simulink model "Implantation_Cmd_MCC_PI"  (R2018b)
settings: Solver=ode1  StartTime=0.0  StopTime=15  FixedStep=Te1  RelTol=1e-3  EnableMultiTasking=on
values from neighbouring files (symbols this model uses):
  Te1 = 0.002    [InitCommande_Aero.m]    (also in matlab_variables_2_2.mat)
undefined symbols (not defined in the file or in its folder): Kpw, Tiw
libraries: quanser_aero x1, simulink_extras x1
settings Model: SimulationMode=external  ExtModeTrigDuration=50000  Creator=MLevis  LastModifiedBy=ACS3
settings SolverCC: PositivePriorityOrder=on
settings DataIOCC: SaveFormat=Array  DSMLogging=off
settings OptimizationCC: LifeSpan=inf
settings DebuggingCC: SolverPrmCheckMsg=warning  SFUnexpectedBacktrackingDiag=warning  SFNoUnconditionalDefaultTransitionDiag=warning  SFExecutionAtInitializationDiag=none
settings HardwareCC: ProdBitPerPointer=32  ProdBitPerSizeT=32  ProdBitPerPtrDiffT=32  ProdLargestAtomicFloat=None  ProdIntDivRoundTo=Undefined  ProdEndianess=Unspecified  ProdWordSize=32  ProdHWDeviceType=32-bit Generic
settings ModelReferenceCC: PropagateSignalLabelsOutOfModel=off
settings SFSimCC: SimUseLocalCustomCode=off
settings RTWCC: SystemTargetFile=quarc_win64.tlc  TemplateMakefile=quarc_default_tmf  Description=QUARC Win64 Target  RTWUseLocalCustomCode=off
settings CodeAppCC: StateflowObjectComments=on
settings STFCustomTargetCC: TargetPreCompLibLocation=C:\PROGRA~3\QUARC\lib\2018b\win64\release  ConcurrentExecutionCompliant=on  GeneratePreprocessorConditionals=Disable all  GRTInterface=on  SystemTargetFile=quarc_win64.tlc
settings GRTTargetCC: TargetPreCompLibLocation=C:\PROGRA~3\QUARC\lib\2018b\win64\release  TargetLangStandard=C89/C90 (ANSI)  ParMdlRefBuildCompliant=off  CompOptLevelCompliant=off  GeneratePreprocessorConditionals=Disable all  CombineOutputUpdateFcns=off  MatFileLogging=off  CPPClassGenCompliant=off  GRTInterface=on  UseToolchainInfoCompliant=off  ExtMode=on  ExtModeMexFile=quarc_comm
settings ConfigComp: CovMetricSettings=dw  CovHtmlReporting=on  CovSaveCumulativeToWorkspaceVar=on  CovSaveSingleToWorkspaceVar=on  CovExternalEMLEnable=off  CovSFcnEnable=off

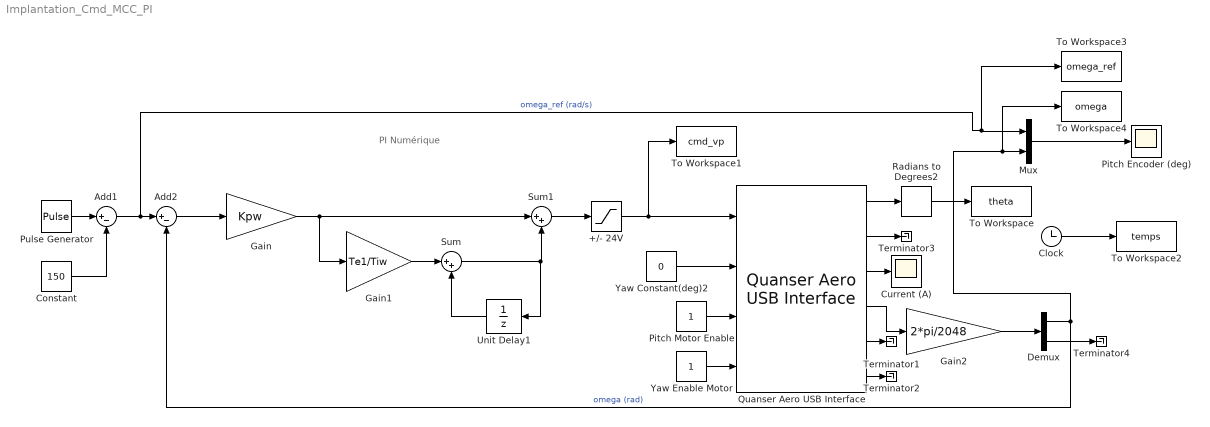
== system Implantation_Cmd_MCC_PI ==
  note: PI Numérique
  +/- 24V : Saturate  UpperLimit=24  LowerLimit=-24
  Add1 : Sum  Inputs=|+-
  Add2 : Sum  Inputs=|+-
  Clock : Clock
  Constant : Constant  Value=150
  Current (A) : Scope
  Demux : Demux  Outputs=2
  Gain : Gain  Gain=Kpw
  Gain1 : Gain  Gain=Te1/Tiw
  Gain2 : Gain  Gain=2*pi/2048
  Mux : Mux  Inputs=2
  Pitch Encoder (deg) : Scope
  Pitch Motor Enable : Constant
  Pulse Generator : DiscretePulseGenerator  PulseType=Time based  Amplitude=150*2  Period=6  PulseWidth=50
  Quanser Aero USB Interface : quanser_aero/Quanser Aero USB Interface  SystemSampleTime=-1
  Radians to Degrees2 : simulink_extras/Transformations/Radians to Degrees
  Sum : Sum  Inputs=|++
  Sum1 : Sum  Inputs=|++
  Terminator{1..4} (4 alike) : Terminator
  To Workspace : ToWorkspace  VariableName=theta  SampleTime=-1
      settings: Save2DSignal=2-D array (concatenate along first dimension)
  To Workspace1 : ToWorkspace  VariableName=cmd_vp  SampleTime=-1
      settings: Save2DSignal=2-D array (concatenate along first dimension)
  To Workspace2 : ToWorkspace  VariableName=temps  SampleTime=-1
      settings: Save2DSignal=2-D array (concatenate along first dimension)
  To Workspace3 : ToWorkspace  VariableName=omega_ref  SampleTime=-1
      settings: Save2DSignal=2-D array (concatenate along first dimension)
  To Workspace4 : ToWorkspace  VariableName=omega  SampleTime=-1
      settings: Save2DSignal=2-D array (concatenate along first dimension)
  Unit Delay1 : UnitDelay  SampleTime=Te1
  Yaw Constant(deg)2 : Constant  Value=0
  Yaw Enable Motor : Constant
  wires:
  Mux/1 -> Pitch Encoder (deg)/1
  Pitch Motor Enable/1 -> Quanser Aero USB Interface/3
  Yaw Enable Motor/1 -> Quanser Aero USB Interface/4
  +/- 24V/1 -> Quanser Aero USB Interface/1, To Workspace1/1
  Quanser Aero USB Interface/3 -> Current (A)/1
  Quanser Aero USB Interface/1 -> Radians to Degrees2/1
  Quanser Aero USB Interface/4 -> Gain2/1
  Quanser Aero USB Interface/5 -> Terminator1/1
  Quanser Aero USB Interface/6 -> Terminator2/1
  Yaw Constant(deg)2/1 -> Quanser Aero USB Interface/2
  Radians to Degrees2/1 -> To Workspace/1
  Quanser Aero USB Interface/2 -> Terminator3/1
  Pulse Generator/1 -> Add1/1
  Clock/1 -> To Workspace2/1
  Constant/1 -> Add1/2
  Gain1/1 -> Sum/1
  Unit Delay1/1 -> Sum/2
  Sum1/1 -> +/- 24V/1
  Gain/1 -> Sum1/1, Gain1/1
  Add2/1 -> Gain/1
  Add1/1 -> To Workspace3/1, Mux/1, Add2/1  "omega_ref (rad/s)"
  Sum/1 -> Unit Delay1/1, Sum1/2
  Gain2/1 -> Demux/1
  Demux/2 -> Terminator4/1
  Demux/1 -> Add2/2, To Workspace4/1, Mux/2  "omega (rad)"
